simulink model "turbulence_DrydenModel"  (R2014a)
settings: Solver=ode45  StartTime=0.0  StopTime=10  MaxStep=0.01  RelTol=1e-3
values from neighbouring files (symbols this model uses):
  turbolenceParameters = initTurbulenceParameters(h,turbolenceParameters,severityChoosed)    [comparingModels.m]
  Va = input('Choose aircraft airspeed [m/s]\nVa=')    [comparingModels.m]
libraries: simulink x1
settings Model: Creator=Domenico  LastModifiedBy=Domenico

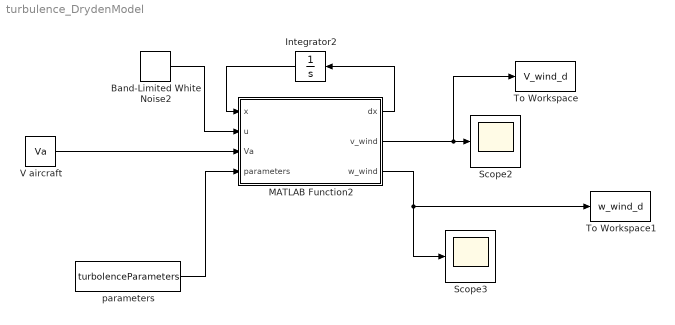
== system turbulence_DrydenModel ==
  Band-Limited White Noise2 : simulink/Sources/Band-Limited White Noise  Cov=[0.1]  Ts=0.1  seed=[23341]
  Integrator2 : Integrator  InitialCondition=zeros(12,1)'
  MATLAB Function2 : MATLAB Function  TreatAsAtomicUnit=on
  Scope2 : Scope
      settings: ShowLegends=on
  Scope3 : Scope
      settings: ShowLegends=on  SaveName=ScopeData3
  To Workspace : ToWorkspace  VariableName=V_wind_d  SaveFormat=Structure With Time  SampleTime=-1
  To Workspace1 : ToWorkspace  VariableName=w_wind_d  SaveFormat=Structure With Time  SampleTime=-1
  V aircraft : Constant  Value=Va
  parameters : Constant  Value=turbolenceParameters  OutDataTypeStr=Bus: myParamsType
  wires:
  Integrator2/1 -> MATLAB Function2/1(x)
  MATLAB Function2/1(dx) -> Integrator2/1
  Band-Limited White Noise2/1 -> MATLAB Function2/2(u)
  V aircraft/1 -> MATLAB Function2/3(Va)
  MATLAB Function2/3(w_wind) -> Scope3/1, To Workspace1/1
  MATLAB Function2/2(v_wind) -> To Workspace/1, Scope2/1
  parameters/1 -> MATLAB Function2/4(parameters)

== matlab function turbulence_DrydenModel/MATLAB Function2 ==
  data: x input; u input; dx output; v_wind output; w_wind output; Va input; parameters input
function [dx,v_wind,w_wind]  = fcn(x,u,Va,parameters)
%This function returns V_wind and w_wind vectors by linear and angular
%velocity of wind - Dryden Model

%   Form: fcn(x,u,parameters,V)
%   Inputs :    x              -> state
%               u              -> white noise
%               parameters     -> vector parameters
%               V              -> velocity aircraft
%   Outputs :   V_wind         -> linear speed wind [u,v,w]
%               w_wind         -> angular rate wind [p,q,r]
%               dx             -> differential state

%% State component
ux   = x(1); % longitudinal u-component (TRANSLATIONAL COMPONENT)
vx   = x(2); % lateral v-component (TRANSLATIONAL COMPONENT)
vxd  = x(3); % derived v-component
wx   = x(4); % vertical w-component(TRANSLATIONAL COMPONENT)
wxd  = x(5); % derived w-component
px   = x(6); % Longitudinal p-component (ROTATIONAL COMPONENT)
rx   = x(7); % Lateral r-component (ROTATIONAL COMPONENT)
rxd  = x(8); % derived of r-component
rx2d = x(9); % second derived of r-component
qx   = x(10);% vertical q-component (ROTATIONAL COMPONENT)
qxd  = x(11);% derived of p-component
qx2d = x(12);% second derived of p-component

%% Input 
eta = u; % white noise

%% Parameters
%turbolence intensities
sigma_u = parameters.sigma_u;
sigma_v = parameters.sigma_v;
sigma_w = parameters.sigma_w;
%scale lengths
Lu      = parameters.Lu;
Lv      = parameters.Lv;
Lw      = parameters.Lw;
b       = parameters.b; %wing span

%% Util terms
bTerm = Lu/Va;
aTerm = sigma_u*sqrt((2*bTerm)/pi);
dTerm = Lv/Va;
cTerm = sigma_v*sqrt(dTerm/pi);
fTerm = Lw/Va; 
eTerm = sigma_v*sqrt(fTerm/pi);
gTerm = (sigma_w*sqrt(0.8/Va)*(pi/(4*b)^(1/6)))/(Lw^(1/3));
hTerm = (4*b)/(pi*Va);
iTerm = (3*b)/(pi*Va);

dx=[-ux/bTerm + eta;
   vxd;
   -(vx/(dTerm^2)) - (2*vxd/dTerm) + eta;
   wxd;
   -wx/(fTerm^2)-(2*wxd)/fTerm+eta;
   -px/hTerm+eta;
   rxd;
   rx2d;
   -rx/(dTerm^2*iTerm)-((2*dTerm+iTerm)/(dTerm^2*iTerm))*rxd-((dTerm^2+2*dTerm*iTerm)/(dTerm^2*iTerm))*rx2d+eta;
   qxd;
   qx2d;
   -qx/(fTerm^2*hTerm)-((2*fTerm+hTerm)/(fTerm^2*hTerm))*qxd-((fTerm^2+2*fTerm*hTerm)/(fTerm^2*hTerm))*qx2d+eta;
];

%% Translational component of wind 
ugw = aTerm/bTerm*ux;                                     % Longitudinal
vgw = (cTerm/(dTerm^2))*vx+(sqrt(3)/dTerm)*cTerm*vxd;     % Lateral
wgw = eTerm/(fTerm^2)*wx+sqrt(3)/fTerm*eTerm*wxd;         % Vertical

%% Rotational component of wind 
pgw = gTerm/hTerm*px;                                                       % Longitudinal
rgw = cTerm/(dTerm^2*iTerm*Va)*rxd+(sqrt(3)*cTerm)/(dTerm*iTerm*Va)*rx2d;   % Lateral
qgw = eTerm/(fTerm^2*hTerm*Va)*qxd+(sqrt(3)*eTerm)/(fTerm*hTerm*Va)*qx2d;   % Vertical

v_wind=[ugw;vgw;wgw];
w_wind=[pgw;qgw;rgw];
    
end
